simulink model "LPV"  (R2013a)
settings: Solver=ode45  StartTime=0.0  StopTime=10.0  RelTol=1e-3
values from neighbouring files (symbols this model uses):
  G = P*B    [Init.m]
  H = -pinv(C*E)*E    [Init.m]
  L = K-N*H    [Init.m]
  N = P*A-K*C    [Init.m]
settings Model: Creator=Ömer  LastModifiedBy=Ömer

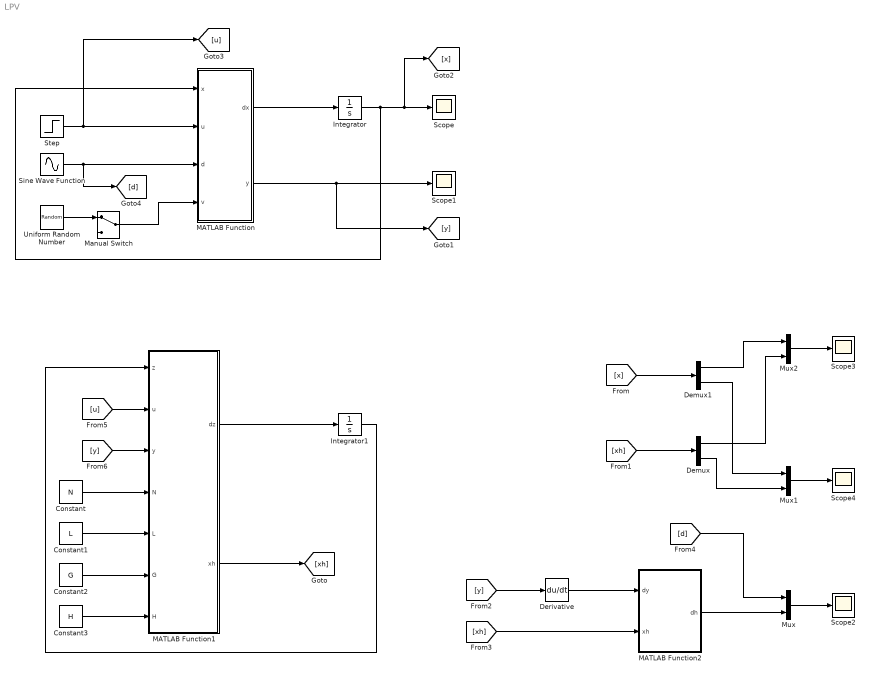
== system LPV ==
  Constant : Constant  Value=N
  Constant1 : Constant  Value=L
  Constant2 : Constant  Value=G
  Constant3 : Constant  Value=H
  Demux : Demux  Outputs=2
  Demux1 : Demux  Outputs=2
  Derivative : Derivative
  Integrator : Integrator  InitialCondition=[1 0]
  Integrator1 : Integrator  InitialCondition=[1 1]
  MATLAB Function : MATLAB Function  TreatAsAtomicUnit=on
  MATLAB Function1 : MATLAB Function  TreatAsAtomicUnit=on
  MATLAB Function2 : MATLAB Function  TreatAsAtomicUnit=on
  Manual Switch : ManualSwitch
  Mux : Mux  Inputs=2
  Mux1 : Mux  Inputs=2
  Mux2 : Mux  Inputs=2
  Scope{,1..4} (5 alike) : Scope
      Scope settings: TimeRange=10
      Scope2 settings: SaveName=ScopeData2
      Scope3 settings: SaveName=ScopeData3
      Scope4 settings: SaveName=ScopeData4
  Sine Wave Function : Sin  SampleTime=0
  Step : Step  Time=5  SampleTime=0
  Uniform Random Number : UniformRandomNumber  Minimum=-.1  Maximum=.1  SampleTime=0.01
  wires:
  Step/1 -> [u], MATLAB Function/2(u)
  Sine Wave Function/1 -> [d], MATLAB Function/3(d)
  Manual Switch/1 -> MATLAB Function/4(v)
  Uniform Random Number/1 -> Manual Switch/1
  MATLAB Function/1(dx) -> Integrator/1
  Integrator/1 -> MATLAB Function/1(x), [x], Scope/1
  Constant/1 -> MATLAB Function1/4(N)
  Constant1/1 -> MATLAB Function1/5(L)
  Constant2/1 -> MATLAB Function1/6(G)
  Constant3/1 -> MATLAB Function1/7(H)
  MATLAB Function1/1(dz) -> Integrator1/1
  Integrator1/1 -> MATLAB Function1/1(z)
  Derivative/1 -> MATLAB Function2/1(dy)
  MATLAB Function/2(y) -> [y], Scope1/1
  MATLAB Function2/1(dh) -> Mux/2
  Mux/1 -> Scope2/1
  Mux1/1 -> Scope4/1
  Mux2/1 -> Scope3/1
  Demux1/1 -> Mux2/1
  Demux/1 -> Mux2/2
  Demux1/2 -> Mux1/1
  Demux/2 -> Mux1/2
  [x] -> Demux1/1
  [xh] -> Demux/1
  [d] -> Mux/1
  [y] -> Derivative/1
  [xh] -> MATLAB Function2/2(xh)
  [u] -> MATLAB Function1/2(u)
  [y] -> MATLAB Function1/3(y)
  MATLAB Function1/2(xh) -> [xh]

== matlab function LPV/MATLAB Function1 ==
  data: z input; u input; y input; N input; L input; G input; H input; dz output; xh output
function [dz,xh] = fcn(z,u,y,N,L,G,H)
%#codegen
dz = zeros(2,1);


dz = N*z+G*u+L*y;
xh = z-H*y;

== matlab function LPV/MATLAB Function ==
  data: x input; dx output; u input; y output; d input; v input
function [dx,y] = fcn(x,u,d,v)
%#codegen
dx = zeros(2,1);
A = [0 1;-1 -2];
B = [0;1];
E = [1;0];
C = [1 0];

dx = A*x+B*u+E*d;
y = C*x+v;

== matlab function LPV/MATLAB Function2 ==
  data: dy input; dh output; xh input
function dh = fcn(dy,xh)
%#codegen
A = [0 1;-1 -2];
B = [0;1];
E = [1;0];
C = [1 0];

dh = pinv(C*E)*(dy-C*A*xh);
